simulink model "CD"  (R2025b)
settings: Solver=VariableStepAuto  StartTime=0.0  StopTime=50  RelTol=1e-3
libraries: commdigbbndpm3 x4, commchan3 x2, commsink2 x2, commblkcod2 x2, commrandsrc3 x1
settings Model: NumberOfSteps=20

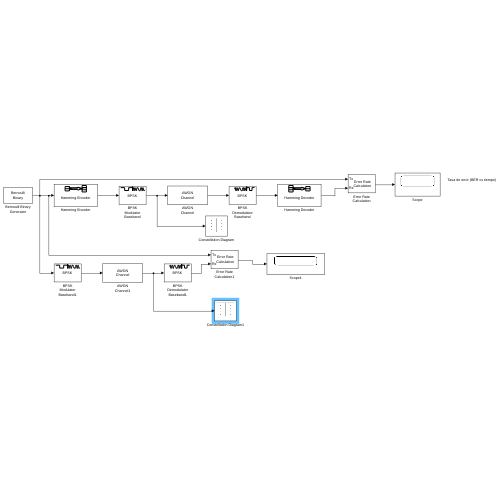
[thumbnail: Simulink's stored preview of the top-level diagram]
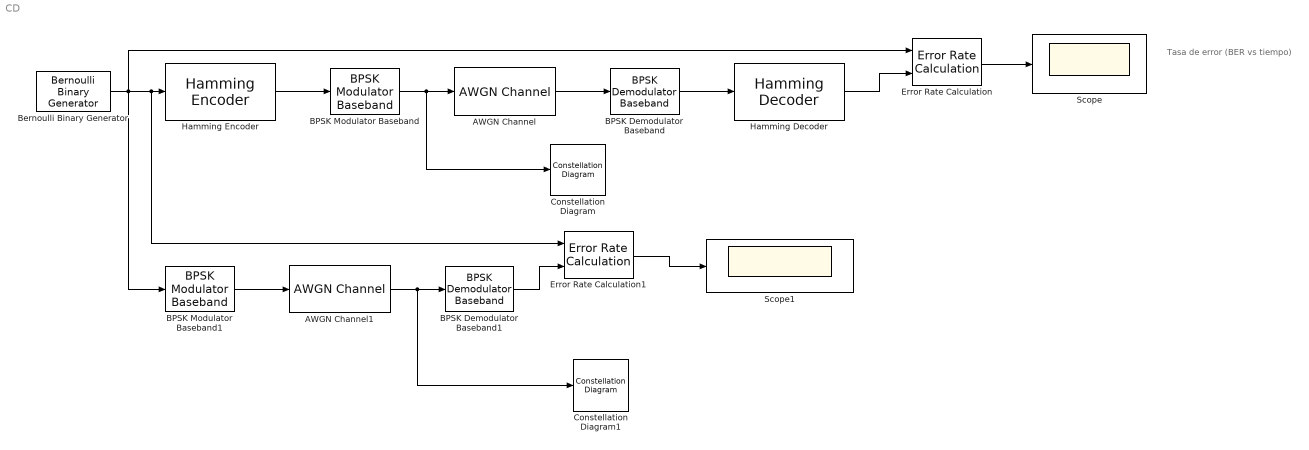
== system CD ==
  note: Tasa de error (BER vs tiempo)
  AWGN Channel : commchan3/AWGN Channel  LegacyMode=off  NoiseMethod="Signal to noise ratio  (SNR)"  noiseMode="Signal to noise ratio  (SNR)"  EbNo=10  EsNo=10  SNR=0  BitsPerSymbol=1  SignalPower=1  SpecifySymbolPeriod=off  SamplesPerSymbol=1  SymbolPeriod=1  VarianceSource=Parameter  Variance=1  RandomStream=mt19937ar with seed  Seed=54321  SimulateUsing=Code generation
  AWGN Channel1 : commchan3/AWGN Channel  LegacyMode=off  NoiseMethod="Signal to noise ratio  (SNR)"  noiseMode="Signal to noise ratio  (SNR)"  EbNo=10  EsNo=10  SNR=0  BitsPerSymbol=1  SignalPower=1  SpecifySymbolPeriod=off  SamplesPerSymbol=1  SymbolPeriod=1  VarianceSource=Parameter  Variance=1  RandomStream=mt19937ar with seed  Seed=54321  SimulateUsing=Code generation
  BPSK Demodulator Baseband : commdigbbndpm3/BPSK Demodulator Baseband  DecType=Hard decision  VarSource=Dialog  Variance=1  Ph=0  outDtype=uint8  derotateFactorWordLen=16  derotateFactorDataTypeStr=Inherit: Same word length as input  derotateFactorLastDataTypeStr=Inherit: Same word length as input
  BPSK Demodulator Baseband1 : commdigbbndpm3/BPSK Demodulator Baseband  DecType=Hard decision  VarSource=Dialog  Variance=1  Ph=0  outDtype=uint8  derotateFactorWordLen=16  derotateFactorDataTypeStr=Inherit: Same word length as input  derotateFactorLastDataTypeStr=Inherit: Same word length as input
  BPSK Modulator Baseband : commdigbbndpm3/BPSK Modulator Baseband  Ph=0  outDtype=single  outWordLen=16  outUDDataType=sfix(16)  outFracLenMode=Best precision  outFracLen=15  outDataTypeStr=single  outLastDataTypeStr=single
  BPSK Modulator Baseband1 : commdigbbndpm3/BPSK Modulator Baseband  Ph=0  outDtype=single  outWordLen=16  outUDDataType=sfix(16)  outFracLenMode=Best precision  outFracLen=15  outDataTypeStr=single  outLastDataTypeStr=single
  Bernoulli Binary Generator : commrandsrc3/Bernoulli Binary Generator  ProbabilityOfZero=0.5  SeedSource=Parameter  Seed=12345  SampleTime=0.001  SamplesPerFrame=4  OutputDataType=uint8  SimulateUsing=Interpreted execution
  Constellation Diagram : ConstellationDiagram  WindowPosition=[1195.000000,1.000000,342.000000,712.000000,]  Visible=on  ContainerLayout="{\"WindowBounds\":[1195,1418,340,710]}"
  Constellation Diagram1 : ConstellationDiagram  Visible=on  ContainerLayout="{\"WindowBounds\":[1,1419,1534,709]}"
  Error Rate Calculation : commsink2/Error Rate Calculation  N=0  st_delay=0  cp_mode=Entire frame  subframe=[]  PMode=Port  WsName=ErrorVec  RsMode2=off  stop=on  numErr=100  maxBits=1e6
  Error Rate Calculation1 : commsink2/Error Rate Calculation  N=0  st_delay=0  cp_mode=Entire frame  subframe=[]  PMode=Port  WsName=ErrorVec  RsMode2=off  stop=on  numErr=100  maxBits=1e6
  Hamming Decoder : commblkcod2/Hamming Decoder  n=7  k=4
  Hamming Encoder : commblkcod2/Hamming Encoder  n=7  k=4
  Scope : Scope
      settings: RequirementInfo="{}  %GIDa_73bb534b_b2ea_4ca4_a718_d04fc26a29f3"  ActiveDisplayYMinimum=-124291.99999999997  ActiveDisplayYMaximum=1.118628E+6
  Scope1 : Scope
      settings: ActiveDisplayYMinimum=-124950.99999999997  ActiveDisplayYMaximum=1.124559E+6
  wires:
  Bernoulli Binary Generator/1 -> Error Rate Calculation1/1, Hamming Encoder/1, BPSK Modulator Baseband1/1, Error Rate Calculation/1
  Hamming Encoder/1 -> BPSK Modulator Baseband/1
  BPSK Modulator Baseband/1 -> Constellation Diagram/1, AWGN Channel/1
  AWGN Channel/1 -> BPSK Demodulator Baseband/1
  BPSK Demodulator Baseband/1 -> Hamming Decoder/1
  Hamming Decoder/1 -> Error Rate Calculation/2
  Error Rate Calculation/1 -> Scope/1
  BPSK Modulator Baseband1/1 -> AWGN Channel1/1
  AWGN Channel1/1 -> Constellation Diagram1/1, BPSK Demodulator Baseband1/1
  BPSK Demodulator Baseband1/1 -> Error Rate Calculation1/2
  Error Rate Calculation1/1 -> Scope1/1
